simulink model "advanced_robotics_control"  (R2024a)
settings: Solver=ode1  StartTime=0.0  StopTime=10.0  FixedStep=0.01  RelTol=1e-3
settings Model: Creator=gujun  LastModifiedBy=jun
settings RTWCC: GPUComputeCapability=3.5

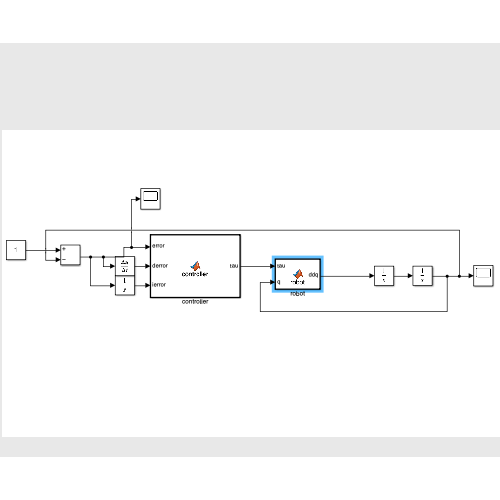
[thumbnail: Simulink's stored preview of the top-level diagram]
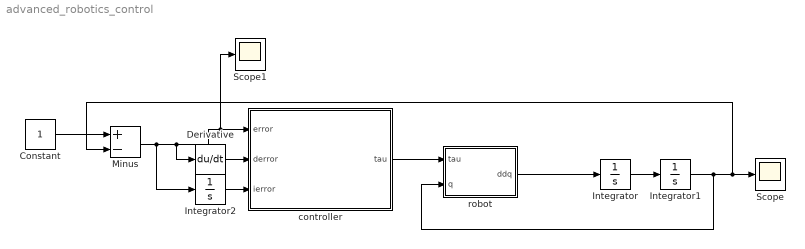
== system advanced_robotics_control ==
  Constant : Constant
  Derivative : Derivative
  Integrator : Integrator
  Integrator1 : Integrator
  Integrator2 : Integrator
  Minus : Sum  Inputs=+-
  Scope : Scope
  Scope1 : Scope
  controller : MATLAB Function  TreatAsAtomicUnit=on
  robot : MATLAB Function  TreatAsAtomicUnit=on
  wires:
  controller/1(tau) -> robot/1(tau)
  robot/1(ddq) -> Integrator/1
  Integrator/1 -> Integrator1/1
  Integrator1/1 -> robot/2(q), Minus/2, Scope/1
  Constant/1 -> Minus/1
  Minus/1 -> Integrator2/1, Derivative/1, Scope1/1, controller/1(error)
  Integrator2/1 -> controller/3(ierror)
  Derivative/1 -> controller/2(derror)

== matlab function advanced_robotics_control/controller ==
  data: error input; tau output; derror input; ierror input
function tau = controller(error, derror, ierror)

kp = 8;

ki = 5;

kd = 0.7;

tau = kp * error + kd * derror + ki * ierror;

== matlab function advanced_robotics_control/robot ==
  data: tau input; ddq output; q input
function ddq = robot(tau, q)

I = 0.01;

m = 0.5;

lg = 0.2;

g = 9.8;
% g = 0;
Ibar = I + m * lg * lg;

tauBar = tau - m * g * lg * cos(q);

ddq = tauBar / Ibar;
